simulink model "Plant_Model"  (R2024b)
settings: Solver=FixedStepDiscrete  StartTime=0.0  StopTime=10.0  FixedStep=50e-6  RelTol=1e-3
values from neighbouring files (symbols this model uses):
  p = 4    [PID_Data.m]    (also in PMSM_PID_Data.m)
  Ts = 1/20000    (= 5e-05)    [PID_Data.m]    (also in PMSM_PID_Data.m)
  Vdc = 300    [PID_Data.m]    (also in PMSM_PID_Data.m = 40)
libraries: mcbplantlib x1, autolibpmsmexterior x1
settings Model: Creator=BitCore  LastModifiedBy=BitCore

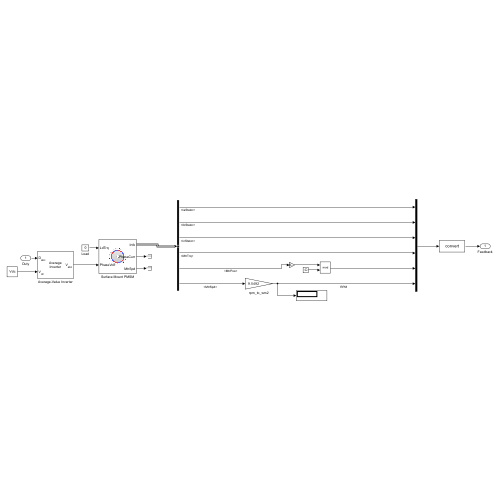
[thumbnail: Simulink's stored preview of the top-level diagram]
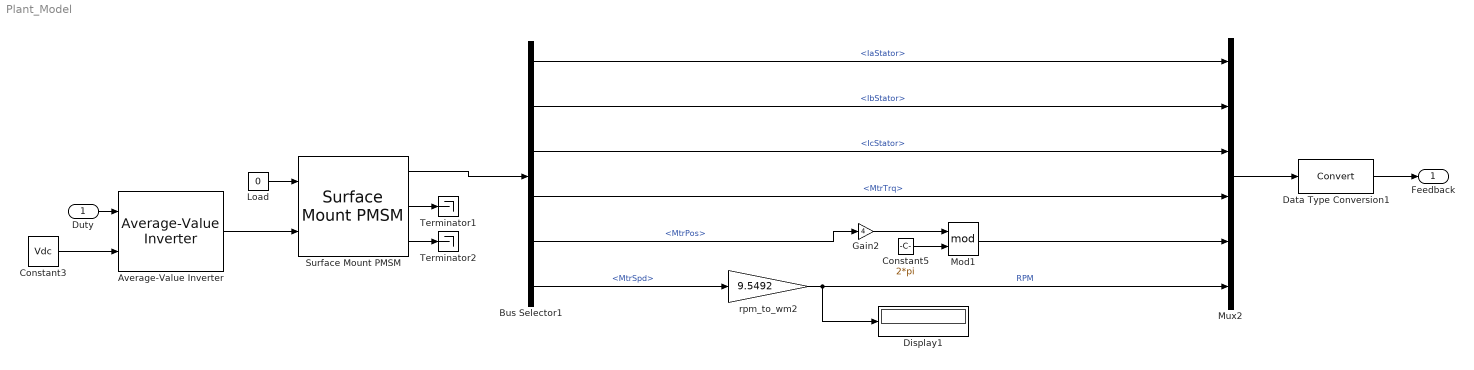
== system Plant_Model ==
  Duty : Inport
  Average-Value Inverter : mcbplantlib/Average-Value Inverter
      settings: LibrarySourceBlock=mcblib/Electrical Systems/Inverters/Average-Value Inverter
  Bus Selector1 : BusSelector  OutputSignals=IaStator,IbStator,IcStator,MtrTrq,MtrPos,MtrSpd
  Constant3 : Constant  Value=Vdc
  Constant5 : Constant  Value=2*pi
  Data Type Conversion1 : DataTypeConversion  SaturateOnIntegerOverflow=off  RndMeth=Floor
  Display1 : Display
  Gain2 : Gain  Gain=4
  Load : Constant  Value=0
  Mod1 : Math  Operator=mod
  Mux2 : Mux  Inputs=6
  Surface Mount PMSM : autolibpmsmexterior/Surface Mount PMSM  port_config=Torque  sim_type=Discrete  Ts=Ts  P=p  Rs=Rs  Ldq_=Ld  KConstText=Permanent flux linkage constant (lambda_pm):  lambda_pm=Lambda  Ke=159.9771  Kt=1.323  mechanical=[0.0027 0.0004924 4 ]  idq0=[0 0]  theta_init=0  omega_init=0  KConst=Lambda  lambda_pm_calc=Lambda  RefBlkName='autolibpmsmexterior/Surface Mount PMSM'  aMode=5  Ldq="[0.0017      0.0017]"
  Terminator1 : Terminator
  Terminator2 : Terminator
  rpm_to_wm2 : Gain  Gain=9.5492  OutDataTypeStr=double
  Feedback : Outport  OutDataTypeStr=single
  wires:
  Constant3/1 -> Average-Value Inverter/2
  Average-Value Inverter/1 -> Surface Mount PMSM/2
  Duty/1 -> Average-Value Inverter/1
  Load/1 -> Surface Mount PMSM/1
  Surface Mount PMSM/1 -> Bus Selector1/1
  Surface Mount PMSM/2 -> Terminator1/1
  Surface Mount PMSM/3 -> Terminator2/1
  Data Type Conversion1/1 -> Feedback/1
  Gain2/1 -> Mod1/1
  Bus Selector1/3 -> Mux2/3  "<IcStator>"
  Bus Selector1/5 -> Gain2/1  "<MtrPos>"
  Bus Selector1/1 -> Mux2/1  "<IaStator>"
  Bus Selector1/2 -> Mux2/2  "<IbStator>"
  Mux2/1 -> Data Type Conversion1/1
  Bus Selector1/4 -> Mux2/4  "<MtrTrq>"
  Constant5/1 -> Mod1/2
  rpm_to_wm2/1 -> Mux2/6, Display1/1  "RPM"
  Mod1/1 -> Mux2/5
  Bus Selector1/6 -> rpm_to_wm2/1  "<MtrSpd>"
